simulink model "testMomentumObserverWithDataFromExperiments"  (R2020a)
settings: Solver=VariableStepAuto  StartTime=0.0  StopTime=nrOfSamples  RelTol=1e-3
undefined symbols (not defined in the file): nrOfJoints
settings Model: Creator=iiticublap041  LastModifiedBy=iiticublap041

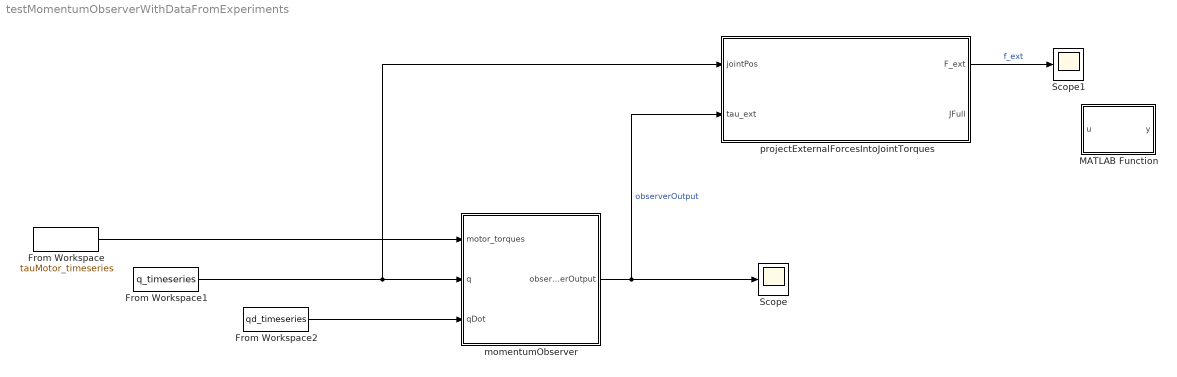
== system testMomentumObserverWithDataFromExperiments ==
  From Workspace : FromWorkspace  VariableName=tauMotor_timeseries
  From Workspace1 : FromWorkspace  VariableName=q_timeseries
  From Workspace2 : FromWorkspace  VariableName=qd_timeseries
  MATLAB Function : MATLAB Function  TreatAsAtomicUnit=on
  Scope : Scope
  Scope1 : Scope
  momentumObserver : Subsystem
  projectExternalForcesIntoJointTorques : MATLAB Function  TreatAsAtomicUnit=on
  wires:
  From Workspace/1 -> momentumObserver/1(motor_torques)
  From Workspace1/1 -> projectExternalForcesIntoJointTorques/1(jointPos), momentumObserver/2(q)
  From Workspace2/1 -> momentumObserver/3(qDot)
  momentumObserver/1(observerOutput) -> projectExternalForcesIntoJointTorques/2(tau_ext), Scope/1  "observerOutput"
  projectExternalForcesIntoJointTorques/1(F_ext) -> Scope1/1  "f_ext"

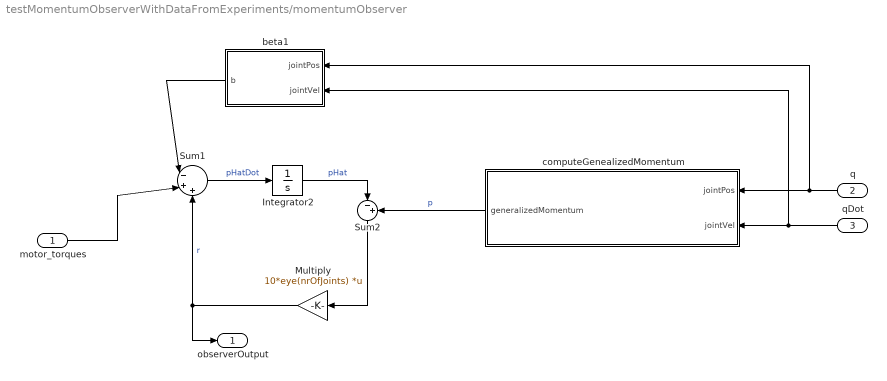
== system testMomentumObserverWithDataFromExperiments/momentumObserver ==
  motor_torques : Inport
  q : Inport  Port=2
  qDot : Inport  Port=3
  Integrator2 : Integrator
  Multiply : Gain  Gain=10*eye(nrOfJoints)  Multiplication=Matrix(K*u) (u vector)
  Sum1 : Sum  Inputs=|-++
  Sum2 : Sum  Inputs=|-+
  beta1 : MATLAB Function  TreatAsAtomicUnit=on
  computeGenealizedMomentum : MATLAB Function  TreatAsAtomicUnit=on
  observerOutput : Outport
  wires:
  Sum1/1 -> Integrator2/1  "pHatDot"
  Multiply/1 -> Sum1/3, observerOutput/1  "r"
  computeGenealizedMomentum/1(generalizedMomentum) -> Sum2/2  "p"
  beta1/1(b) -> Sum1/1
  Sum2/1 -> Multiply/1
  Integrator2/1 -> Sum2/1  "pHat"
  motor_torques/1 -> Sum1/2
  qDot/1 -> beta1/2(jointVel), computeGenealizedMomentum/2(jointVel)
  q/1 -> computeGenealizedMomentum/1(jointPos), beta1/1(jointPos)

== matlab function testMomentumObserverWithDataFromExperiments/projectExternalForcesIntoJointTorques ==
  data: jointPos input; F_ext output; tau_ext input; JFull output
function [F_ext,JFull] = projectExternalForcesIntoJointTorques(jointPos,tau_ext)

% Use rnea mex function
coder.extrinsic('computeNumericalJacobian');
J = computeNumericalJacobian('computeNumericalJacobian',jointPos);
% Assign the output to a vaiable of known type.
% See https://www.mathworks.com/help/simulink/ug/calling-matlab-functions.html#bq1h2z9-47
F_ext = zeros(6,1);
JFull = zeros(max(size(jointPos)));
JFull = full(J);
F_ext = ((JFull.')^-1)*tau_ext;
end

== matlab function testMomentumObserverWithDataFromExperiments/MATLAB Function ==
  data: u input; y output
function y = determinant(u)

y = det(u);

== matlab function testMomentumObserverWithDataFromExperiments/momentumObserver/beta1 ==
  data: jointPos input; b output; jointVel input
function b = beta(jointPos,jointVel)
% Compute gravity torques using RNEA with appropriate inputs
qd_grav = 0;
qdd = 0;
F_ext = 0;
% TODO: do not hard code gravity 
g = [0;0;-9.81];
coder.extrinsic('rnea');
tau_gravity = rnea('rnea',jointPos,qd_grav,qdd,g,F_ext);
% Assign the output to a vaiable of kwown type.
% See https://www.mathworks.com/help/simulink/ug/calling-matlab-functions.html#bq1h2z9-47
tau_gravityFull = zeros(max(size(jointPos,1)),1);
tau_gravityFull = full(tau_gravity);
% Coriolis matrix
coder.extrinsic('computeCoriolisMatrix');
C = computeCoriolisMatrix('computeCoriolisMatrix',jointPos,jointVel);
CFull = zeros(max(size(jointPos,1)));
CFull = full(C);
b = tau_gravityFull - CFull.'*jointVel;

== matlab function testMomentumObserverWithDataFromExperiments/momentumObserver/computeGenealizedMomentum ==
  data: jointPos input; jointVel input; generalizedMomentum output
function generalizedMomentum = computeGeneralizedMomentum(jointPos,jointVel)
coder.extrinsic('computeMassMatrix'); 
M = computeMassMatrix('computeMassMatrix', jointPos);
% Assign the output to a vaiable of kwown type.
% See https://www.mathworks.com/help/simulink/ug/calling-matlab-functions.html#bq1h2z9-47
MFull = zeros(max(size(jointPos)));
MFull = full(M);
generalizedMomentum = MFull*jointVel;
